simulink model "Helical_Traj_HeadlessPositionControllerVariableQuadDynamicsMdl"  (R2016b)
settings: Solver=FixedStepAuto  StartTime=0.0  StopTime=25  FixedStep=0.1  RelTol=1e-3  EnableMultiTasking=on
undefined symbols (not defined in the file): Params, QuaternionController_lqr, traj_helix, TrajControl_LQR
settings Model: Creator=Raj  LastModifiedBy=CDSLAB-User
settings DataIOCC: LimitDataPoints=on  SaveFormat=Array
settings OptimizationCC: LifeSpan=inf
settings DebuggingCC: UnderspecifiedInitializationDetection=Classic  MergeDetectMultiDrivingBlocksExec=none  SolverPrmCheckMsg=warning  StateNameClashWarn=warning  SFUnexpectedBacktrackingDiag=warning  SFNoUnconditionalDefaultTransitionDiag=warning  SFExecutionAtInitializationDiag=none
settings HardwareCC: ProdBitPerPointer=32  ProdBitPerSizeT=32  ProdBitPerPtrDiffT=32  ProdLargestAtomicFloat=None  ProdIntDivRoundTo=Undefined  ProdEndianess=Unspecified  ProdWordSize=32  ProdHWDeviceType=32-bit Generic
settings ModelReferenceCC: PropagateSignalLabelsOutOfModel=off
settings GRTTargetCC: TargetLangStandard=C89/C90 (ANSI)  GeneratePreprocessorConditionals=Disable all
settings ConfigComp: CovMetricSettings=dw  CovHtmlReporting=on  CovSaveCumulativeToWorkspaceVar=on  CovSaveSingleToWorkspaceVar=on  CovExternalEMLEnable=off  CovSFcnEnable=off

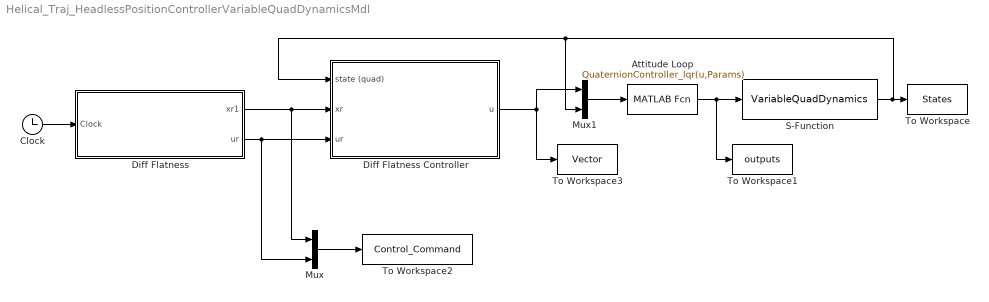
== system Helical_Traj_HeadlessPositionControllerVariableQuadDynamicsMdl ==
  Attitude Loop : MATLABFcn  MATLABFcn=QuaternionController_lqr(u,Params)  OutputDimensions=4
  Clock : Clock
      settings: Decimation=100
  Diff Flatness : Subsystem
  Diff Flatness Controller : Subsystem
  Mux : Mux  Inputs=2
  Mux1 : Mux  Inputs=2
  S-Function : S-Function  FunctionName=VariableQuadDynamics  Parameters=Params  SFunctionDeploymentMode=off  EnableBusSupport=off
  To Workspace : ToWorkspace  VariableName=States  SaveFormat=Timeseries  SampleTime=-1
  To Workspace1 : ToWorkspace  VariableName=outputs  SaveFormat=Timeseries  SampleTime=-1
  To Workspace2 : ToWorkspace  VariableName=Control_Command  SaveFormat=Timeseries  SampleTime=-1
  To Workspace3 : ToWorkspace  VariableName=Vector  SaveFormat=Timeseries  SampleTime=-1
  wires:
  Attitude Loop/1 -> S-Function/1, To Workspace1/1
  S-Function/1 -> To Workspace/1, Diff Flatness Controller/1(state (quad)), Mux1/2
  Mux1/1 -> Attitude Loop/1
  Diff Flatness Controller/1(u) -> To Workspace3/1, Mux1/1
  Clock/1 -> Diff Flatness/1("Clock ")
  Diff Flatness/1(xr1) -> Mux/1, Diff Flatness Controller/2("xr ")
  Diff Flatness/2(ur) -> Mux/2, Diff Flatness Controller/3(ur)
  Mux/1 -> To Workspace2/1

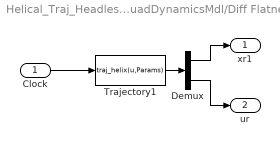
== system Helical_Traj_HeadlessPositionControllerVariableQuadDynamicsMdl/Diff Flatness ==
  "Clock " : Inport
  Demux : Demux  Outputs=2
  Trajectory1 : MATLABFcn  MATLABFcn=traj_helix(u,Params)  OutputDimensions=12
  xr1 : Outport
  ur : Outport  Port=2  PortDimensions=4
  wires:
  "Clock "/1 -> Trajectory1/1
  Trajectory1/1 -> Demux/1
  Demux/1 -> xr1/1
  Demux/2 -> ur/1

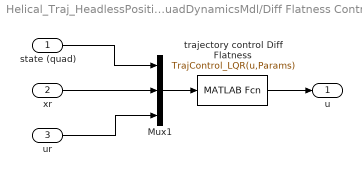
== system Helical_Traj_HeadlessPositionControllerVariableQuadDynamicsMdl/Diff Flatness Controller ==
  state (quad) : Inport
  "xr " : Inport  Port=2
  ur : Inport  Port=3
  Mux1 : Mux  Inputs=3
  trajectory control Diff Flatness : MATLABFcn  MATLABFcn=TrajControl_LQR(u,Params)  OutputDimensions=4
  u : Outport
  wires:
  trajectory control Diff Flatness/1 -> u/1
  state (quad)/1 -> Mux1/1
  Mux1/1 -> trajectory control Diff Flatness/1
  ur/1 -> Mux1/3
  "xr "/1 -> Mux1/2
